simulink model "control"  (R2022b)
settings: Solver=VariableStepAuto  StartTime=0.0  StopTime=4  RelTol=1e-3
undefined symbols (not defined in the file or in its folder): DiscIntNeverNeededParam
libraries: matrix_library x2
settings Model: Creator=giuseppeloianno  LastModifiedBy=brigh
settings DataIOCC: ReturnWorkspaceOutputs=off

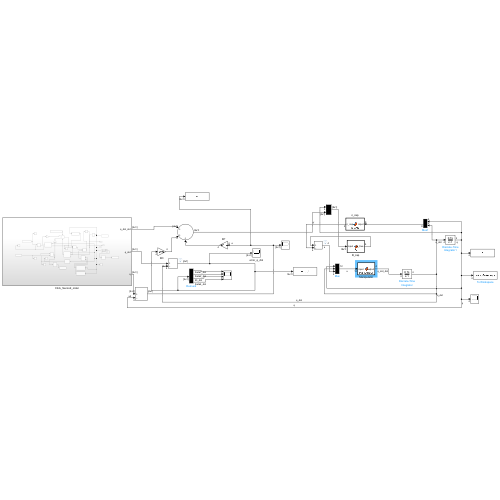
[thumbnail: Simulink's stored preview of the top-level diagram]
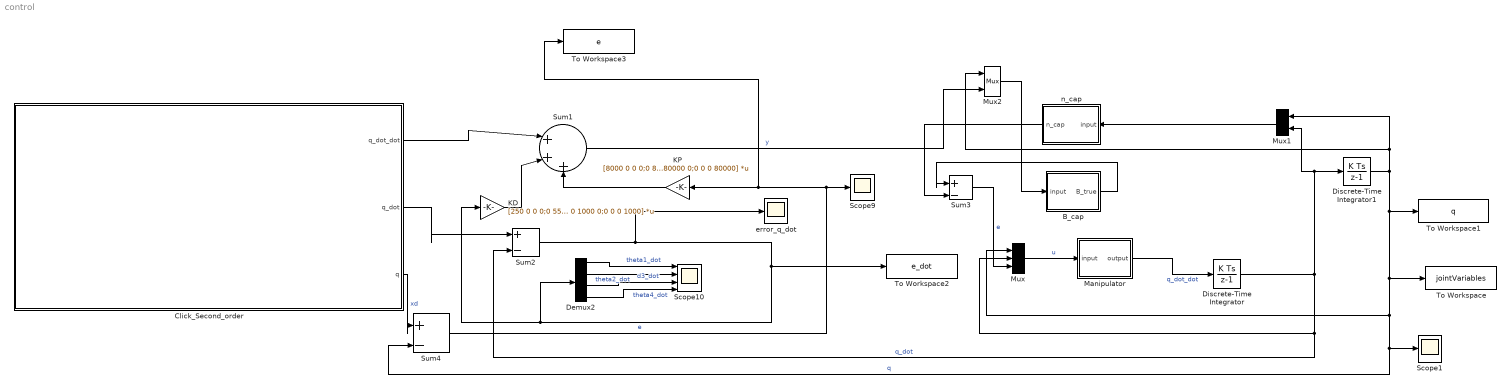
== system control ==
  B_cap : MATLAB Function  TreatAsAtomicUnit=on
  Click_Second_order : Subsystem
  Demux2 : Demux
  Discrete-Time Integrator : DiscreteIntegrator  InitialCondition=[0;0;0;0]  SampleTime=0.001  ICPrevOutput=DiscIntNeverNeededParam  ICPrevScaledInput=DiscIntNeverNeededParam
  Discrete-Time Integrator1 : DiscreteIntegrator  InitialCondition=[-0.9273;-1.2870;0.700;2.2143]  SampleTime=0.001  ICPrevOutput=DiscIntNeverNeededParam  ICPrevScaledInput=DiscIntNeverNeededParam
  KD : Gain  Gain=[250 0 0 0;0 550 0 0;0 0 1000 0;0 0 0 1000]  Multiplication=Matrix(K*u) (u vector)
  KP : Gain  Gain=[8000 0 0 0;0 8000 0 0;0 0 80000 0;0 0 0 80000]  Multiplication=Matrix(K*u) (u vector)
  Manipulator : MATLAB Function  TreatAsAtomicUnit=on
  Mux : Mux  Inputs=3
  Mux1 : Mux  Inputs=2
  Mux2 : Mux  Inputs=2
  Scope1 : Scope
  Scope10 : Scope  NumInputPorts=4
  Scope9 : Scope
  Sum1 : Sum  Inputs=|+++
  Sum2 : Sum  Inputs=|+-
  Sum3 : Sum  Inputs=|+-
  Sum4 : Sum  Inputs=|+-
  To Workspace : ToWorkspace  VariableName=jointVariables  SampleTime=-1
  To Workspace1 : ToWorkspace  VariableName=q  SampleTime=-1
  To Workspace2 : ToWorkspace  VariableName=e_dot  SampleTime=-1
  To Workspace3 : ToWorkspace  VariableName=e  SampleTime=-1
  error_q_dot : Scope
  n_cap : MATLAB Function  TreatAsAtomicUnit=on
  wires:
  Mux/1 -> Manipulator/1(input)  "u"
  Demux2/1 -> Scope10/1  "theta1_dot"
  n_cap/1(n_cap) -> Sum3/2
  Sum1/1 -> Mux2/2  "y"
  B_cap/1(B_true) -> Sum3/1
  Demux2/2 -> Scope10/2  "theta2_dot"
  Sum2/1 -> To Workspace2/1, Demux2/1, KD/1, error_q_dot/1
  Discrete-Time Integrator1/1 -> Mux2/1, Mux1/1, Sum4/2, Scope1/1, Mux/1, To Workspace/1, To Workspace1/1  "q"
  Mux1/1 -> n_cap/1(input)
  Demux2/3 -> Scope10/3  "d3_dot"
  Manipulator/1(output) -> Discrete-Time Integrator/1  "q_dot_dot"
  Discrete-Time Integrator/1 -> Sum2/2, Mux/2, Mux1/2, Discrete-Time Integrator1/1  "q_dot"
  KD/1 -> Sum1/2
  Click_Second_order/3(q) -> Sum4/1  "xd"
  Sum3/1 -> Mux/3  "e"
  Click_Second_order/2(q_dot) -> Sum2/1
  Sum4/1 -> Scope9/1, To Workspace3/1, KP/1  "e"
  Mux2/1 -> B_cap/1(input)
  Demux2/4 -> Scope10/4  "theta4_dot"
  Click_Second_order/1(q_dot_dot) -> Sum1/1
  KP/1 -> Sum1/3

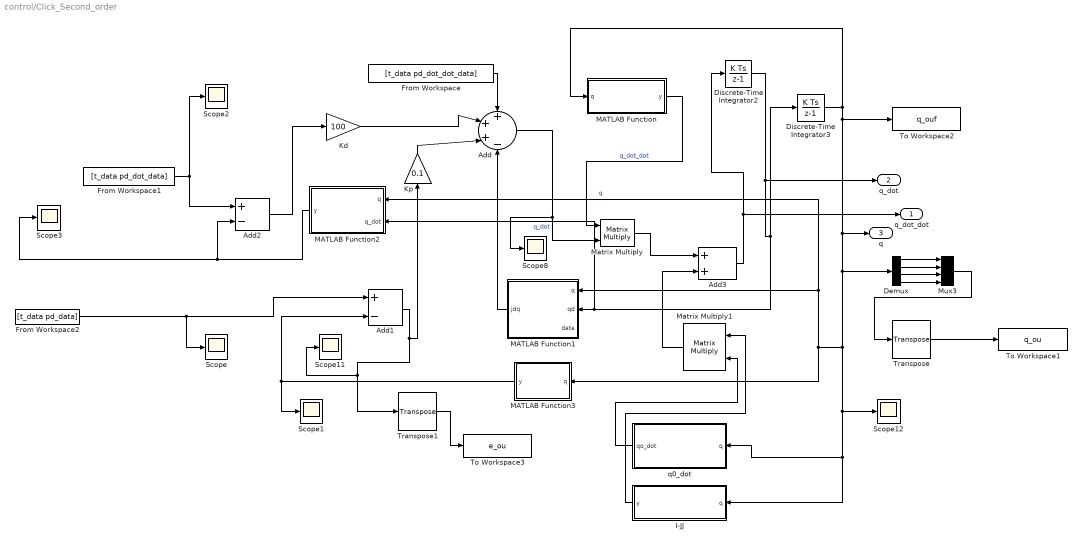
== system control/Click_Second_order ==
  Add : Sum  Inputs=+++-
  Add1 : Sum  Inputs=+-
  Add2 : Sum  Inputs=+-
  Add3 : Sum
  Demux : Demux
  Discrete-Time Integrator2 : DiscreteIntegrator  InitialCondition=[-0.927293431584587;-1.287005790420619;0.700000000000000;2.214299222005206]  SampleTime=0.001  LimitOutput=on  UpperSaturationLimit=[pi/2 pi/4 1 2*pi]'  LowerSaturationLimit="[-pi/2 -pi/2 0.25  -2*pi]'"  ICPrevOutput=DiscIntNeverNeededParam  ICPrevScaledInput=DiscIntNeverNeededParam
  Discrete-Time Integrator3 : DiscreteIntegrator  InitialCondition=[-0.9273;-1.2870;0.700;2.2143]  SampleTime=0.001  LimitOutput=on  UpperSaturationLimit=[pi/2 pi/4 1 2*pi]'  LowerSaturationLimit="[-pi/2 -pi/2 0.25  -2*pi]'"  ICPrevOutput=DiscIntNeverNeededParam  ICPrevScaledInput=DiscIntNeverNeededParam
  From Workspace : FromWorkspace  VariableName=[t_data pd_dot_dot_data]  SampleTime=0.001
  From Workspace1 : FromWorkspace  VariableName=[t_data pd_dot_data]  SampleTime=0.001
  From Workspace2 : FromWorkspace  VariableName=[t_data pd_data]  SampleTime=0.001
  I-JJ : MATLAB Function  TreatAsAtomicUnit=on
  Kd : Gain  Gain=100
  Kp : Gain  Gain=0.1
  MATLAB Function : MATLAB Function  TreatAsAtomicUnit=on
  MATLAB Function1 : MATLAB Function  TreatAsAtomicUnit=on
  MATLAB Function2 : MATLAB Function  TreatAsAtomicUnit=on
  MATLAB Function3 : MATLAB Function  TreatAsAtomicUnit=on
  Matrix Multiply : Product  Multiplication=Matrix(*)
  Matrix Multiply1 : Product  Multiplication=Matrix(*)
  Mux3 : Mux
  Scope{,1..3,8,11..12} (7 alike) : Scope
  To Workspace1 : ToWorkspace  VariableName=q_ou  SampleTime=-1
      settings: Save2DSignal=2-D array (concatenate along first dimension)
  To Workspace2 : ToWorkspace  VariableName=q_ouf  SampleTime=-1
  To Workspace3 : ToWorkspace  VariableName=e_ou  SampleTime=-1
      settings: Save2DSignal=2-D array (concatenate along first dimension)
  Transpose : matrix_library/Transpose
  Transpose1 : matrix_library/Transpose
  q0_dot : MATLAB Function  TreatAsAtomicUnit=on
  q_dot_dot : Outport
  q_dot : Outport  Port=2
  q : Outport  Port=3
  wires:
  Demux/1 -> Mux3/1
  From Workspace/1 -> Add/1
  Demux/2 -> Mux3/2
  Matrix Multiply1/1 -> Add3/2
  Discrete-Time Integrator2/1 -> MATLAB Function2/2(q_dot), MATLAB Function1/2(qd), Discrete-Time Integrator3/1, q_dot/1  "q_dot"
  I-JJ/1(y) -> Matrix Multiply1/1
  MATLAB Function1/1(jdq) -> Add/4
  Add2/1 -> Kd/1
  Kd/1 -> Add/2
  Demux/3 -> Mux3/3
  Matrix Multiply/1 -> Add3/1
  Discrete-Time Integrator3/1 -> Demux/1, Scope12/1, I-JJ/1(q), q0_dot/1(q), MATLAB Function2/1(q), MATLAB Function1/1(q), MATLAB Function3/1(q), q/1, To Workspace2/1, MATLAB Function/1(q)  "q"
  Add1/1 -> Scope11/1, Transpose1/1, Kp/1
  MATLAB Function/1(y) -> Matrix Multiply/1  "q_dot_dot"
  MATLAB Function2/1(y) -> Scope3/1, Add2/2
  From Workspace1/1 -> Add2/1, Scope2/1
  From Workspace2/1 -> Add1/1, Scope/1
  Add/1 -> Matrix Multiply/2, Scope8/1
  Kp/1 -> Add/3
  Add3/1 -> q_dot_dot/1, Discrete-Time Integrator2/1
  MATLAB Function3/1(y) -> Scope1/1, Add1/2
  Mux3/1 -> Transpose/1
  Transpose1/1 -> To Workspace3/1
  Transpose/1 -> To Workspace1/1
  Demux/4 -> Mux3/4
  q0_dot/1(qo_dot) -> Matrix Multiply1/2

== matlab function control/Click_Second_order/MATLAB Function ==
  data: q input; y output
function y =pinvj(q)

a1 = 0.5;
a2 = 0.5;
t1 = q(1);
t2 = q(2);
d3 = q(3);
b = t1+t2;
c1 = cos(t1);
s1 = sin(t1);
c12 = cos(b);
s12 = sin(b);

J = [-a2*s12-a1*s1 -a2*s12 0 0; a2*c12+a1*c1 a2*c12 0 0;  0 0 1 0];
x= pinv(J);
y=x;
end

== matlab function control/Click_Second_order/MATLAB Function2 ==
  data: q input; q_dot input; y output
function y = jacobian(q, q_dot)
a1 = 0.5;
a2 = 0.5;
t1 = q(1);
t2 = q(2);
d3 = q(3);
b = t1+t2;
c1 = cos(t1);
s1 = sin(t1);
c12 = cos(b);
s12 = sin(b);


J = [-a2*s12-a1*s1 -a2*s12 0 0; a2*c12+a1*c1 a2*c12 0 0; 0 0 -1.5+d3 0];
y = J*q_dot;

end

== matlab function control/Click_Second_order/MATLAB Function3 ==
  data: q input; y output
function y = direct_kin(q)
a1=0.5;
a2=0.5;
t1=q(1);
t2=q(2);
b=t1+t2;
d3=q(3);
c1= cos(t1);
s1 = sin(t1);
c12 = cos(b);
s12 = sin(b);
y=[a2*c12+a1*c1;a1*s12+a1*s1;-1.5+d3];
end

== matlab function control/Click_Second_order/I-JJ ==
  data: q input; y output
function y = ijj(q)


a1 = 0.5;
a2 = 0.5;
t1 = q(1);
t2 = q(2);
d3 = q(3);
b = t1+t2;
c1 = cos(t1);
s1 = sin(t1);
c12 = cos(b);
s12 = sin(b);
k = 10;

J = [-a2*s12-a1*s1 -a2*s12 0 0; a2*c12+a1*c1 a2*c12 0 0;0 0 1 0];
x= pinv(J);


c = [1 0 0 0; 0 1 0 0; 0 0 1 0; 0 0 0 1] - (x * J);

p=[0.4;-0.7;0.5;1];


q_dot=[-(2*(sin(b)/2 + sin(q(1))/2)*(cos(b)/2 + cos(q(1))/2 - p(1,:)) - 2*(cos(b)/2 + cos(q(1))/2)*(sin(b)/2 + sin(q(1))/2 + p(2,:)))/(2*((cos(b)/2 + cos(q(1))/2 - p(1,:))^2 + (sin(b)/2 + sin(q(1))/2 + p(2,:))^2 + (q(3) - p(3,:))^2)^(1/2)),  -(sin(b)*(cos(b)/2 + cos(q(1))/2 - p(1,:)) - cos(b)*(sin(b)/2 + sin(q(1))/2 + p(2,:)))/(2*((cos(b)/2 + cos(q(1))/2 - p(1,:))^2 + (sin(b)/2 + sin(q(1))/2 + p(2,:))^2 + (q(3) - p(3,:))^2)^(1/2)),  (2*q(3) - 1)/(2*((cos(b)/2 + cos(q(1))/2 - p(1,:))^2 + (sin(b)/2 + sin(q(1))/2 + p(2,:))^2 + (q(3) - p(3,:))^2)^(1/2)), 0];


g =k* q_dot.';

y = c ;
end

== matlab function control/Click_Second_order/q0_dot ==
  data: q input; qo_dot output
function qo_dot = qodot(q)


a1 = 0.5;
a2 = 0.5;
t1 = q(1);
t2 = q(2);
t3 = q(3);
b = t1+t2;
c1 = cos(t1);
s1 = sin(t1);
c12 = cos(b);
s12 = sin(b);
k = 10;

J = [-a2*s12-a1*s1 -a2*s12 0 0; a2*c12+a1*c1 a2*c12 0 0; 1 1 0 1];
x= pinv(J);


c = [1 0 0 0; 0 1 0 0; 0 0 1 0; 0 0 0 1] - (x * J);

p=[0.4;-0.7;0.5;1];
p1= p(1);
p2=p(2);
p3=p(3);

qo_dot=k * [(-q(1)/(4*(pi)^2));(-4/(9*(pi)^2))*(q(2)+(pi*8));(0.625-q(3))/2.25;-q(4)/(16*(pi)^2)];

end

== matlab function control/B_cap ==
  data: input input; B_true output
function  B_true = B(input)
    theta2=input(2,:);
    y1=input(5,:);
    y2=input(6,:);
    y3=input(7,:);    
    y4=input(8,:);
    ml1 = 25;
    ml2 = 25;
    ml3 = 10;
    ml4 = 0;
    Il1 = 5;
    Il2 = 5;
    Il4 = 1;
    Im1 = 0.0001;
    Im2 = 0.0001;
    Im3 = 0.01;
    Im4 = 0.005;
    l1 = 0.25;
    l2 = 0.25;
    kr1 = 1;
    kr2 = 1;
    kr3 = 50;
    kr4 = 20;
    g = 9.8;

    b11=l1^2*ml1+(0.25+l2^2+l2*cos(theta2))*ml2+(0.5+0.5*cos(theta2))*(ml3+ml4)+Il1+Il2+Il4+Im1*kr1^2+Im2+Im3+Im4;
    b12=(0.5*l2*cos(theta2)+l2^2)*ml2+(0.25+0.25*cos(theta2))*(ml3+ml4)+Il2+Il4+Im2*kr2++Im3+Im4;
    b13=-kr3*Im3;
    b14=kr4*Im4+Il4;
    b21=b12;
    b22=l2^2*ml2+0.25*(ml4+ml3)+Il2+Il4+Im2*kr2^2+Im4+Im3;
    b23=-kr3*Im3;
    b24=kr4*Im4+Il4;
    b31=b13;
    b32=b23;
    b33=Im3*kr3^2+ml3+ml4;
    b34=0;
    b41=b14;
    b42=b24;
    b43=b34;
    b44=Im4*kr4^2+Il4;
    B_t=[b11 b12 b13 b14; b21 b22 b23 b24; b31 b32 b33 b34; b41 b42 b43 b44];
    B_true=B_t*transpose([y1 y2 y3 y4]);
end

== matlab function control/Manipulator ==
  data: input input; output output
function output = Manipulator(input)
% Part 2 manipulator
    t1 = input(1,:);
    t2 = input(2,:);
    d3 = input(3,:);
    t4 = input(4,:);
    t1d = input(5,:);
    t2d = input(6,:);
    d3 = input(7,:);
    t4d = input(8,:);
    u1 = input(9,:);
    u2 = input(10,:);
    u3 = input(11,:);
    u4 = input(12,:);
    ml1 = 25;
    ml2 = 25;
    ml3 = 10;
    ml4 = 5;
    Il1 = 5;
    Il2 = 5;
    Il4 = 1;
    Im1 = 0.0001;
    Im2 = 0.0001;
    Im3 = 0.01;
    Im4 = 0.005;
    l1 = 0.25;
    l2 = 0.25;
    kr1 = 1;
    kr2 = 1;
    kr3 = 50;
    kr4 = 20;
    g = 9.8;
    Fv1 = 0.0001;
    Fv2 = 0.0001;
    Fv3 = 0.01;
    Fv4 = 0.005;
    
    b11=l1^2*ml1+(0.25+l2^2+l2*cos(t2))*ml2+(0.5+0.5*cos(t2))*(ml3+ml4)+Il1+Il2+Il4+Im1*kr1^2+Im2+Im3+Im4;
    b12=(0.5*l2*cos(t2)+l2^2)*ml2+(0.25+0.25*cos(t2))*(ml3+ml4)+Il2+Il4+Im2*kr2++Im3+Im4;
    b13=-kr3*Im3;
    b14=kr4*Im4+Il4;
    b21=b12;
    b22=l2^2*ml2+0.25*(ml4+ml3)+Il2+Il4+Im2*kr2^2+Im4+Im3;
    b23=-kr3*Im3;
    b24=kr4*Im4+Il4;
    b31=b13;
    b32=b23;
    b33=Im3*kr3^2+ml3+ml4;
    b34=0;
    b41=b14;
    b42=b24;
    b43=b34;
    b44=Im4*kr4^2+Il4;
    B=[b11 b12 b13 b14; b21 b22 b23 b24; b31 b32 b33 b34; b41 b42 b43 b44];
    C=[(-l2*ml2*sin(t2)-0.5*(ml4+ml3)*sin(t2))/2*t2d (-l2*ml2*sin(t2)-0.5*(ml4+ml3)*sin(t2))/2*(t1d+t2d) 0 0; -(-l2*ml2*sin(t2)-0.5*(ml4+ml3)*sin(t2))/2*t1d 0 0 0; 0 0 0 0; 0 0 0 0];
    G = [0; 0; -(ml3+ml4)*g; 0];
    
    F = diag([kr1^2*Fv1 kr2^2*Fv2 kr3^2*Fv3 kr4^2*Fv4]);
    
    tou = [u1 u2 u3 u4]';
    tou_1 = C*[t1d t2d d3 t4d]'+F*[t1d t2d d3 t4d]'+G;
    
    q_dot_dot = inv(B)*(tou-tou_1);
    
    output = q_dot_dot;
    
    
    
    
    % output(2) = q_dot_dot(2);
    % output(3) = q_dot_dot(3);
    % output(4) = q_dot_dot(4);
end

== matlab function control/n_cap ==
  data: input input; n_cap output
function n_cap  = n_cap(input)
    t2=input(2,:);
    t1d=input(5,:);
    t2d=input(6,:);
    d3d=input(7,:);
    t4d=input(8,:);
    ml2 = 25;
    ml3 = 10;
    ml4 = 0;
    l2 = 0.25;
    kr1 = 1;
    kr2 = 1;
    kr3 = 50;
    kr4 = 20;
    g = 9.8;
    Fv1 = 0.0001;
    Fv2 = 0.0001;
    Fv3 = 0.01;
    Fv4 = 0.005;
    
    
    Ccap=[(-l2*ml2*sin(t2)-0.5*(ml4+ml3)*sin(t2))/2*t2d (-l2*ml2*sin(t2)-0.5*(ml4+ml3)*sin(t2))/2*(t1d+t2d) 0 0; -(-l2*ml2*sin(t2)-0.5*(ml4+ml3)*sin(t2))/2*t1d 0 0 0; 0 0 0 0; 0 0 0 0];
  
    G = [0; 0; -(ml3+ml4)*g; 0];
    F = diag([kr1^2*Fv1 kr2^2*Fv2 kr3^2*Fv3 kr4^2*Fv4]);
    n_cap = Ccap*[t1d t2d d3d t4d]'+F*[t1d t2d d3d t4d]'+G;
end

== matlab function control/Click_Second_order/MATLAB Function1 ==
  data: q input; qd input; jdq output; data input
function jdq = jacdd(q,qd, data)
t1 = q(1);
t2 = q(2);


t1d = qd(1);
t2d = qd(2);


w = (cos(t1)*t1d)/2;
x = (sin(t1)*t1d)/2;
y = (sin(t1 + t2)*(t1d + t2d))/2;
z = (cos(t1 + t2)*(t1d + t2d))/2;

Jd = [-w-z -z 0 0; -x-y -y 0 0; 0 0 0 0];
jdq = Jd*qd;

end
